simulink model "cv_model_M50"  (R2023a)
settings: Solver=ode23t  StartTime=0  StopTime=700  FixedStep=0.0005  MaxStep=.01  RelTol=1e-4
model workspace (MAT data in the model file):
  test = 0
values from neighbouring files (symbols this model uses):
  A_cheb_09_1 = [-9.45889157397 1 0 0 0 0 0 0 0 -116.684730988 0 1 ... (81 elements, 9x9)]    [input_reflex_filters.mat]
  B_cheb_09_1 = [1 0 0 0 0 0 0 0 0]    [input_reflex_filters.mat]
  C_cheb_09_1 = [0 0 0 0 0 0 0 0 151338.279895]    [input_reflex_filters.mat]
libraries: SignalEditorBlockLib x4, simulink_extras x4
(part 4 of 4)

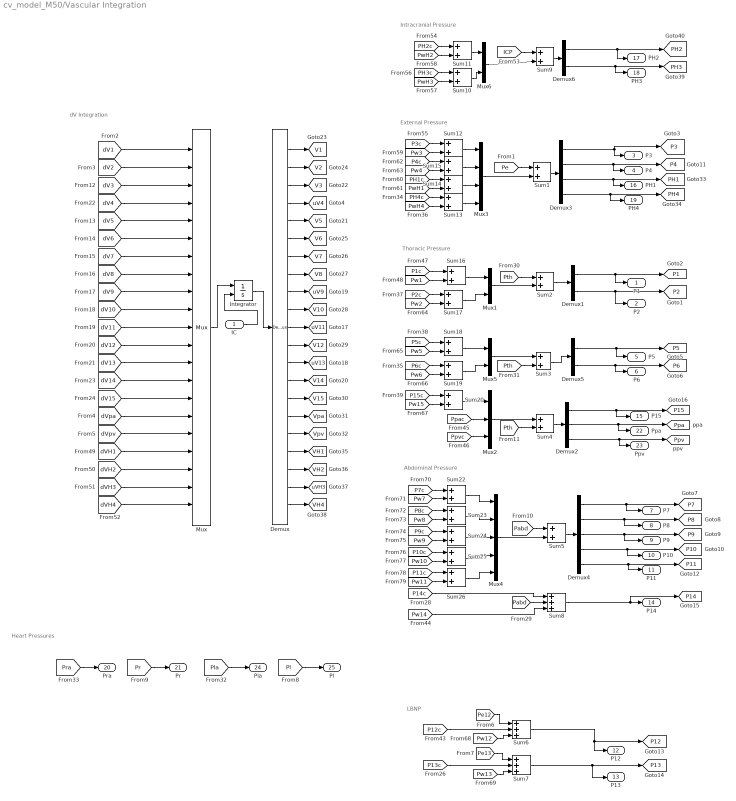
== system cv_model_M50/Vascular Integration ==
  note: Heart Pressures
  note: dV Integration
  note: External Pressure
  note: LBNP
  note: Abdominal Pressure
  note: Thoracic Pressure
  note: Intracranial Pressure
  IC : Inport
  Demux : Demux  Outputs=21
      settings: DisplayOption=none
  Demux1 : Demux  Outputs=2
      settings: DisplayOption=none
  Demux2 : Demux  Outputs=3
      settings: DisplayOption=none
  Demux3 : Demux
      settings: DisplayOption=none
  Demux4 : Demux  Outputs=5
      settings: DisplayOption=none
  Demux5 : Demux  Outputs=2
      settings: DisplayOption=none
  Demux6 : Demux  Outputs=2
      settings: DisplayOption=none
  Integrator : Integrator  InitialConditionSource=external  InitialCondition=[113.4187 4.15 24.2091 19.3527]
  Mux : Mux  Inputs=21
  Mux1 : Mux  Inputs=2
  Mux2 : Mux  Inputs=3
  Mux3 : Mux
  Mux4 : Mux  Inputs=5
  Mux5 : Mux  Inputs=2
  Mux6 : Mux  Inputs=2
  Sum{1..5,9..20,22..26} (22 alike) : Sum  InputSameDT=on  SaturateOnIntegerOverflow=on  OutDataTypeStr=Inherit: Same as first input
  Sum6 : Sum  Inputs=+++  InputSameDT=on  SaturateOnIntegerOverflow=on  OutDataTypeStr=Inherit: Same as first input
  Sum7 : Sum  Inputs=+++  InputSameDT=on  SaturateOnIntegerOverflow=on  OutDataTypeStr=Inherit: Same as first input
  Sum8 : Sum  Inputs=+++  InputSameDT=on  SaturateOnIntegerOverflow=on  OutDataTypeStr=Inherit: Same as first input
  P1 : Outport
  P2 : Outport  Port=2
  P3 : Outport  Port=3
  P4 : Outport  Port=4
  P5 : Outport  Port=5
  P6 : Outport  Port=6
  P7 : Outport  Port=7
  P8 : Outport  Port=8
  P9 : Outport  Port=9
  P10 : Outport  Port=10
  P11 : Outport  Port=11
  P12 : Outport  Port=12
  P13 : Outport  Port=13
  P14 : Outport  Port=14
  P15 : Outport  Port=15
  PH1 : Outport  Port=16
  PH2 : Outport  Port=17
  PH3 : Outport  Port=18
  PH4 : Outport  Port=19
  Pra : Outport  Port=20
  Pr : Outport  Port=21
  Ppa : Outport  Port=22
  Ppv : Outport  Port=23
  Pla : Outport  Port=24
  Pl : Outport  Port=25
  tag scope: P10=global, P11=global, P12=global, P13=global, P14=global, P15=global, P1=global, P2=global, P3=global, P4=global, P5=global, P6=global, P7=global, P8=global, P9=global, PH1=global, PH2=global, PH3=global, PH4=global, Ppa=global, Ppv=global, V10=global, V12=global, V14=global, V15=global, V1=global, V2=global, V3=global, V5=global, V6=global, V7=global, V8=global, VH1=global, VH2=global, VH4=global, Vpa=global, Vpv=global, uV11=global, uV13=global, uV4=global, uV9=global, uVH3=global
  wires:
  [Pl] -> Pl/1
  [Pr] -> Pr/1
  [dV1] -> Mux/1
  [dV2] -> Mux/2
  Demux2/2 -> Ppa/1, [Ppa]
  Demux1/1 -> P1/1, [P1]
  [dVpv] -> Mux/17
  [dVpa] -> Mux/16
  [dV3] -> Mux/3
  [dV4] -> Mux/4
  [dV5] -> Mux/5
  [dV6] -> Mux/6
  [dV7] -> Mux/7
  [dV8] -> Mux/8
  [dV9] -> Mux/9
  [dV10] -> Mux/10
  [dV11] -> Mux/11
  [dV12] -> Mux/12
  [dV13] -> Mux/13
  [dV14] -> Mux/14
  [dV15] -> Mux/15
  Demux1/2 -> [P2], P2/1
  Demux3/1 -> [P3], P3/1
  Demux3/2 -> [P4], P4/1
  Demux5/1 -> [P5], P5/1
  Demux4/1 -> P7/1, [P7]
  Demux4/2 -> P8/1, [P8]
  Demux4/3 -> [P9], P9/1
  Demux4/4 -> P10/1, [P10]
  Demux4/5 -> P11/1, [P11]
  Demux2/1 -> [P15], P15/1
  Demux2/3 -> Ppv/1, [Ppv]
  Demux5/2 -> P6/1, [P6]
  Integrator/1 -> Demux/1
  Mux/1 -> Integrator/1
  IC/1 -> Integrator/2
  [Pth] -> Sum4/2
  Mux1/1 -> Sum2/2
  Sum2/1 -> Demux1/1
  Sum6/1 -> [P12], P12/1
  Sum7/1 -> [P13], P13/1
  Sum8/1 -> [P14], P14/1
  Mux2/1 -> Sum4/1
  Sum4/1 -> Demux2/1
  [Pth] -> Sum2/1
  Demux/4 -> [uV4]
  Mux3/1 -> Sum1/2
  Sum1/1 -> Demux3/1
  [Pe] -> Sum1/1
  [Pth] -> Sum3/2
  [Pabd] -> Sum5/1
  Mux4/1 -> Sum5/2
  Sum5/1 -> Demux4/1
  Mux5/1 -> Sum3/1
  Sum3/1 -> Demux5/1
  [Pe12] -> Sum6/1
  [Pabd] -> Sum8/2
  [Pla] -> Pla/1
  [Pra] -> Pra/1
  Sum15/1 -> Mux3/2
  Demux/13 -> [uV13]
  [P13c] -> Sum7/2
  Demux/9 -> [uV9]
  Sum24/1 -> Mux4/3
  Demux/14 -> [V14]
  [P14c] -> Sum8/1
  Sum18/1 -> Mux5/1
  Demux/5 -> [V5]
  Demux/3 -> [V3]
  Sum12/1 -> Mux3/1
  Demux/1 -> [V1]
  Demux/2 -> [V2]
  Sum16/1 -> Mux1/1
  Sum17/1 -> Mux1/2
  Demux/6 -> [V6]
  Demux/7 -> [V7]
  Demux/8 -> [V8]
  Sum23/1 -> Mux4/2
  Demux/10 -> [V10]
  Demux/12 -> [V12]
  [P12c] -> Sum6/2
  [Pe13] -> Sum7/1
  Demux/15 -> [V15]
  Sum20/1 -> Mux2/1
  Demux/16 -> [Vpa]
  Demux/17 -> [Vpv]
  [Ppac] -> Mux2/2
  [Ppvc] -> Mux2/3
  Demux/11 -> [uV11]
  Sum14/1 -> Mux3/3
  Sum13/1 -> Mux3/4
  Demux3/3 -> [PH1], PH1/1
  Demux3/4 -> [PH4], PH4/1
  [dVH1] -> Mux/18
  [dVH2] -> Mux/19
  [dVH3] -> Mux/20
  [dVH4] -> Mux/21
  Demux/18 -> [VH1]
  Demux/19 -> [VH2]
  Demux/20 -> [uVH3]
  Demux/21 -> [VH4]
  Demux6/1 -> PH2/1, [PH2]
  Mux6/1 -> Sum9/2
  Sum9/1 -> Demux6/1
  [ICP] -> Sum9/1
  Demux6/2 -> PH3/1, [PH3]
  [PH3c] -> Sum10/1
  [PwH3] -> Sum10/2
  Sum10/1 -> Mux6/2
  [PwH2] -> Sum11/2
  [PH2c] -> Sum11/1
  Sum11/1 -> Mux6/1
  [P3c] -> Sum12/1
  [Pw3] -> Sum12/2
  [PH4c] -> Sum13/1
  [PwH4] -> Sum13/2
  [PH1c] -> Sum14/1
  [PwH1] -> Sum14/2
  [P4c] -> Sum15/1
  [Pw4] -> Sum15/2
  [P1c] -> Sum16/1
  [Pw1] -> Sum16/2
  [P2c] -> Sum17/1
  [Pw2] -> Sum17/2
  [P5c] -> Sum18/1
  [Pw5] -> Sum18/2
  [P6c] -> Sum19/1
  [Pw6] -> Sum19/2
  Sum19/1 -> Mux5/2
  [P15c] -> Sum20/1
  [Pw15] -> Sum20/2
  [Pw12] -> Sum6/3
  [Pw13] -> Sum7/3
  [Pw14] -> Sum8/3
  [Pw7] -> Sum22/2
  [P7c] -> Sum22/1
  [Pw8] -> Sum23/2
  [P8c] -> Sum23/1
  [Pw9] -> Sum24/2
  [P9c] -> Sum24/1
  [Pw10] -> Sum25/2
  [P10c] -> Sum25/1
  [Pw11] -> Sum26/2
  [P11c] -> Sum26/1
  Sum22/1 -> Mux4/1
  Sum25/1 -> Mux4/4
  Sum26/1 -> Mux4/5

== system cv_model_M50/Design of Experiment/Switch Block ==
  In1 : Inport
  In2 : Inport  Port=2
  Null Signal : Constant  Value=0
  Switch : Switch  Criteria=u2 > Threshold  Threshold=0.5  SaturateOnIntegerOverflow=off  InputSameDT=off
  Switch Control : Constant
  Switch1 : Switch  Criteria=u2 > Threshold  Threshold=0.5  SaturateOnIntegerOverflow=off  InputSameDT=off
  Tilt Angle : Outport
  Speed : Outport  Port=2
  tag scope: Ctrl=global
  wires:
  Switch Control/1 -> [Ctrl], Switch1/2, Switch/2
  Null Signal/1 -> Switch1/1, Switch/3
  In1/1 -> Switch/1
  Switch/1 -> Tilt Angle/1
  Switch1/1 -> Speed/1
  In2/1 -> Switch1/3
